simulink model "PWMGenerationComponent"  (R2026a)
settings: Solver=FixedStepDiscrete
settings Model: DataDictionary=TractionEmotorSoftwareArchInterfaceData.sldd  Creator=dakaihu  LastModifiedBy=dakaihu

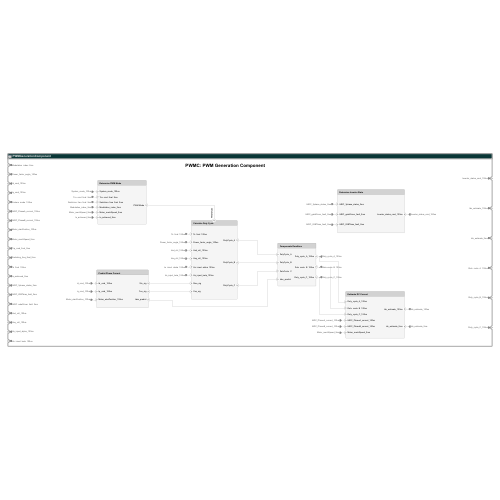
[thumbnail: Simulink's stored preview of the top-level diagram]
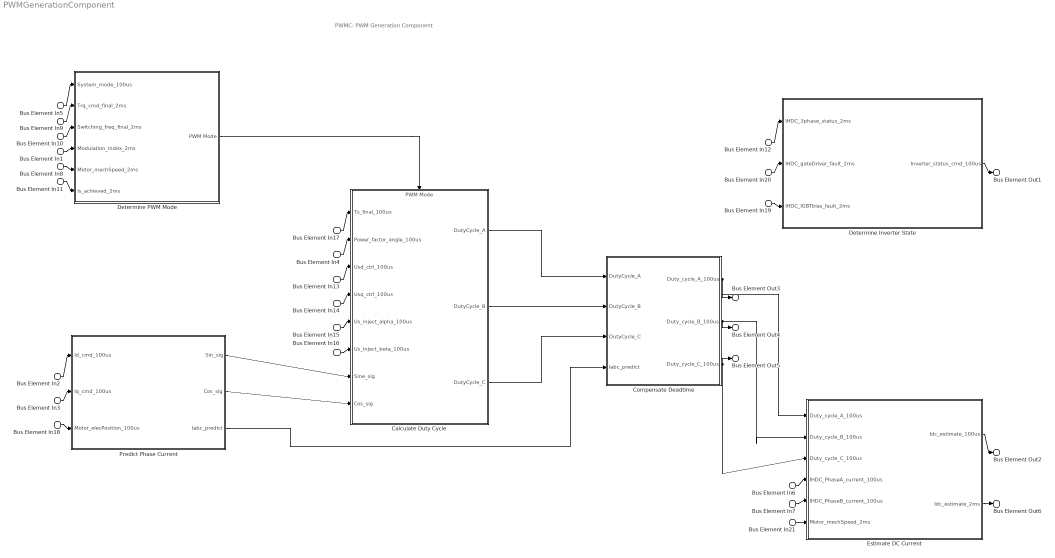
== system PWMGenerationComponent ==
  note: PWMC: PWM Generation Component
  Bus Element In1 : Inport  PortName=Modulation_index_2ms
  Bus Element In4 : Inport  Port=2  PortName=Power_factor_angle_100us
  Bus Element In2 : Inport  Port=3  PortName=Id_cmd_100us
  Bus Element In3 : Inport  Port=4  PortName=Iq_cmd_100us
  Bus Element In5 : Inport  Port=5  PortName=System_mode_100us
  Bus Element In6 : Inport  Port=6  PortName=IHDC_PhaseA_current_100us
  Bus Element In7 : Inport  Port=7  PortName=IHDC_PhaseB_current_100us
  Bus Element In18 : Inport  Port=8  PortName=Motor_elecPosition_100us
  Bus Element In8 : Inport  Port=9  PortName=Motor_mechSpeed_2ms
  Bus Element In21 : Inport  Port=9  PortName=Motor_mechSpeed_2ms
  Bus Element In9 : Inport  Port=10  PortName=Trq_cmd_final_2ms
  Bus Element In10 : Inport  Port=11  PortName=Switching_freq_final_2ms
  Bus Element In17 : Inport  Port=12  PortName=Ts_final_100us
  Bus Element In11 : Inport  Port=13  PortName=Is_achieved_2ms
  Bus Element In12 : Inport  Port=14  PortName=IHDC_3phase_status_2ms
  Bus Element In19 : Inport  Port=15  PortName=IHDC_IGBTbias_fault_2ms
  Bus Element In20 : Inport  Port=16  PortName=IHDC_gateDriver_fault_2ms
  Bus Element In13 : Inport  Port=17  PortName=Usd_ctrl_100us
  Bus Element In14 : Inport  Port=18  PortName=Usq_ctrl_100us
  Bus Element In15 : Inport  Port=19  PortName=Us_inject_alpha_100us
  Bus Element In16 : Inport  Port=20  PortName=Us_inject_beta_100us
  Calculate Duty Cycle : Subsystem
      settings: PortSchema="{\"entries\":[{\"content\":{\"headerSize\":26,\"margin\":15,\"minimumSpacing\":25,\"sides\":[{\"content\":{\"connectorIds\":[\"In2\",\"In3\",\"In4\",\"In5\",\"In6\",\"In7\",\"In8\",\"In9\"]},\"type\":\"ConnectorPlacement.EquallySpacedRectSide\",\"uuid\":\"a0c63ab2-75fe-4bec-b2b0-6e2e00a1a5a4\"},{\"content\":{\"connectorIds\":[\"Out1\",\"Out2\",\"Out3\"],\"side\":\"RIGHT\"},\"type\":\"ConnectorPlacement.EquallySpacedRectSide\",\"uuid\":\"05d605ea-8968-4533-a01c-bf4aae5caa93\"},{\"content\":{\"connectorIds\":[\"In1\"],\"side\":\"TOP\"},\"type\":\"ConnectorPlacement.EquallySpacedRectSide\",\"uuid\":\"27167c69-3967-4107-acce-f317c3d854af\"}]},\"type\":\"ConnectorPlacement.EquallySpacedConnector\",\"uuid\":\"c4d90da2-0f2a-4c00-bd24-85fead00d18f\"}],\"packageUris\":[\"http://schema.mathworks.com/mf0/Connector/R2020b\"],\"version\":\"1.0\"}"
  Compensate Deadtime : Subsystem
      settings: PortSchema="{\"entries\":[{\"content\":{\"headerSize\":26,\"margin\":15,\"minimumSpacing\":25,\"sides\":[{\"content\":{\"connectorIds\":[\"In1\",\"In2\",\"In3\",\"In4\"]},\"type\":\"ConnectorPlacement.EquallySpacedRectSide\",\"uuid\":\"a0c63ab2-75fe-4bec-b2b0-6e2e00a1a5a4\"},{\"content\":{\"connectorIds\":[\"Out1\",\"Out2\",\"Out3\"],\"side\":\"RIGHT\"},\"type\":\"ConnectorPlacement.EquallySpacedRectSide\",\"uuid\":\"05d605ea-8968-4533-a01c-bf4aae5caa93\"},{\"content\":{\"connectorIds\":[],\"side\":\"TOP\"},\"type\":\"ConnectorPlacement.EquallySpacedRectSide\",\"uuid\":\"27167c69-3967-4107-acce-f317c3d854af\"}]},\"type\":\"ConnectorPlacement.EquallySpacedConnector\",\"uuid\":\"c4d90da2-0f2a-4c00-bd24-85fead00d18f\"}],\"packageUris\":[\"http://schema.mathworks.com/mf0/Connector/R2020b\"],\"version\":\"1.0\"}"
  Determine Inverter State : Subsystem
      settings: PortSchema="{\"entries\":[{\"content\":{\"headerSize\":26,\"margin\":15,\"minimumSpacing\":25,\"sides\":[{\"content\":{\"connectorIds\":[\"In1\",\"In2\",\"In3\"]},\"type\":\"ConnectorPlacement.EquallySpacedRectSide\",\"uuid\":\"a0c63ab2-75fe-4bec-b2b0-6e2e00a1a5a4\"},{\"content\":{\"connectorIds\":[\"Out1\"],\"side\":\"RIGHT\"},\"type\":\"ConnectorPlacement.EquallySpacedRectSide\",\"uuid\":\"05d605ea-8968-4533-a01c-bf4aae5caa93\"},{\"content\":{\"connectorIds\":[],\"side\":\"TOP\"},\"type\":\"ConnectorPlacement.EquallySpacedRectSide\",\"uuid\":\"27167c69-3967-4107-acce-f317c3d854af\"}]},\"type\":\"ConnectorPlacement.EquallySpacedConnector\",\"uuid\":\"c4d90da2-0f2a-4c00-bd24-85fead00d18f\"}],\"packageUris\":[\"http://schema.mathworks.com/mf0/Connector/R2020b\"],\"version\":\"1.0\"}"
  Determine PWM Mode : Subsystem
      settings: PortSchema="{\"entries\":[{\"content\":{\"headerSize\":26,\"margin\":15,\"minimumSpacing\":25,\"sides\":[{\"content\":{\"connectorIds\":[\"In1\",\"In2\",\"In3\",\"In4\",\"In5\",\"In6\"]},\"type\":\"ConnectorPlacement.EquallySpacedRectSide\",\"uuid\":\"a0c63ab2-75fe-4bec-b2b0-6e2e00a1a5a4\"},{\"content\":{\"connectorIds\":[\"Out1\"],\"side\":\"RIGHT\"},\"type\":\"ConnectorPlacement.EquallySpacedRectSide\",\"uuid\":\"05d605ea-8968-4533-a01c-bf4aae5caa93\"},{\"content\":{\"connectorIds\":[],\"side\":\"TOP\"},\"type\":\"ConnectorPlacement.EquallySpacedRectSide\",\"uuid\":\"27167c69-3967-4107-acce-f317c3d854af\"}]},\"type\":\"ConnectorPlacement.EquallySpacedConnector\",\"uuid\":\"c4d90da2-0f2a-4c00-bd24-85fead00d18f\"}],\"packageUris\":[\"http://schema.mathworks.com/mf0/Connector/R2020b\"],\"version\":\"1.0\"}"
  Estimate DC Current : Subsystem
      settings: PortSchema="{\"entries\":[{\"content\":{\"headerSize\":26,\"margin\":15,\"minimumSpacing\":25,\"sides\":[{\"content\":{\"connectorIds\":[\"In1\",\"In2\",\"In3\",\"In4\",\"In5\",\"In6\"]},\"type\":\"ConnectorPlacement.EquallySpacedRectSide\",\"uuid\":\"a0c63ab2-75fe-4bec-b2b0-6e2e00a1a5a4\"},{\"content\":{\"connectorIds\":[\"Out1\",\"Out2\"],\"side\":\"RIGHT\"},\"type\":\"ConnectorPlacement.EquallySpacedRectSide\",\"uuid\":\"05d605ea-8968-4533-a01c-bf4aae5caa93\"},{\"content\":{\"connectorIds\":[],\"side\":\"TOP\"},\"type\":\"ConnectorPlacement.EquallySpacedRectSide\",\"uuid\":\"27167c69-3967-4107-acce-f317c3d854af\"}]},\"type\":\"ConnectorPlacement.EquallySpacedConnector\",\"uuid\":\"c4d90da2-0f2a-4c00-bd24-85fead00d18f\"}],\"packageUris\":[\"http://schema.mathworks.com/mf0/Connector/R2020b\"],\"version\":\"1.0\"}"
  Predict Phase Current : Subsystem
      settings: PortSchema="{\"entries\":[{\"content\":{\"headerSize\":26,\"margin\":15,\"minimumSpacing\":25,\"sides\":[{\"content\":{\"connectorIds\":[\"In1\",\"In2\",\"In3\"]},\"type\":\"ConnectorPlacement.EquallySpacedRectSide\",\"uuid\":\"a0c63ab2-75fe-4bec-b2b0-6e2e00a1a5a4\"},{\"content\":{\"connectorIds\":[\"Out1\",\"Out2\",\"Out3\"],\"side\":\"RIGHT\"},\"type\":\"ConnectorPlacement.EquallySpacedRectSide\",\"uuid\":\"05d605ea-8968-4533-a01c-bf4aae5caa93\"},{\"content\":{\"connectorIds\":[],\"side\":\"TOP\"},\"type\":\"ConnectorPlacement.EquallySpacedRectSide\",\"uuid\":\"27167c69-3967-4107-acce-f317c3d854af\"}]},\"type\":\"ConnectorPlacement.EquallySpacedConnector\",\"uuid\":\"c4d90da2-0f2a-4c00-bd24-85fead00d18f\"}],\"packageUris\":[\"http://schema.mathworks.com/mf0/Connector/R2020b\"],\"version\":\"1.0\"}"
  Bus Element Out1 : Outport  PortName=Inverter_status_cmd_100us
  Bus Element Out2 : Outport  Port=2  PortName=Idc_estimate_100us
  Bus Element Out6 : Outport  Port=3  PortName=Idc_estimate_2ms
  Bus Element Out3 : Outport  Port=4  PortName=Duty_cycle_A_100us
  Bus Element Out4 : Outport  Port=5  PortName=Duty_cycle_B_100us
  Bus Element Out5 : Outport  Port=6  PortName=Duty_cycle_C_100us
  wires:
  Bus Element In12/1 -> Determine Inverter State/1(IHDC_3phase_status_2ms)
  Bus Element In20/1 -> Determine Inverter State/2(IHDC_gateDriver_fault_2ms)
  Bus Element In19/1 -> Determine Inverter State/3(IHDC_IGBTbias_fault_2ms)
  Bus Element In2/1 -> Predict Phase Current/1(Id_cmd_100us)
  Bus Element In3/1 -> Predict Phase Current/2(Iq_cmd_100us)
  Bus Element In18/1 -> Predict Phase Current/3(Motor_elecPosition_100us)
  Predict Phase Current/3(Iabc_predict) -> Compensate Deadtime/4(Iabc_predict)
  Predict Phase Current/1(Sin_sig) -> Calculate Duty Cycle/8(Sine_sig)
  Predict Phase Current/2(Cos_sig) -> Calculate Duty Cycle/9(Cos_sig)
  Bus Element In13/1 -> Calculate Duty Cycle/4(Usd_ctrl_100us)
  Bus Element In14/1 -> Calculate Duty Cycle/5(Usq_ctrl_100us)
  Bus Element In15/1 -> Calculate Duty Cycle/6(Us_inject_alpha_100us)
  Bus Element In16/1 -> Calculate Duty Cycle/7(Us_inject_beta_100us)
  Bus Element In4/1 -> Calculate Duty Cycle/3(Power_factor_angle_100us)
  Bus Element In17/1 -> Calculate Duty Cycle/2(Ts_final_100us)
  Bus Element In5/1 -> Determine PWM Mode/1(System_mode_100us)
  Bus Element In9/1 -> Determine PWM Mode/2(Trq_cmd_final_2ms)
  Bus Element In1/1 -> Determine PWM Mode/4(Modulation_index_2ms)
  Bus Element In10/1 -> Determine PWM Mode/3(Switching_freq_final_2ms)
  Bus Element In8/1 -> Determine PWM Mode/5(Motor_mechSpeed_2ms)
  Bus Element In11/1 -> Determine PWM Mode/6(Is_achieved_2ms)
  Determine PWM Mode/1(PWM Mode) -> Calculate Duty Cycle/1(PWM Mode)
  Calculate Duty Cycle/1(DutyCycle_A) -> Compensate Deadtime/1(DutyCycle_A)
  Calculate Duty Cycle/2(DutyCycle_B) -> Compensate Deadtime/2(DutyCycle_B)
  Calculate Duty Cycle/3(DutyCycle_C) -> Compensate Deadtime/3(DutyCycle_C)
  Bus Element In6/1 -> Estimate DC Current/4(IHDC_PhaseA_current_100us)
  Bus Element In7/1 -> Estimate DC Current/5(IHDC_PhaseB_current_100us)
  Bus Element In21/1 -> Estimate DC Current/6(Motor_mechSpeed_2ms)
  Estimate DC Current/1(Idc_estimate_100us) -> Bus Element Out2/1
  Compensate Deadtime/1(Duty_cycle_A_100us) -> Bus Element Out3/1, Estimate DC Current/1(Duty_cycle_A_100us)
  Compensate Deadtime/2(Duty_cycle_B_100us) -> Bus Element Out4/1, Estimate DC Current/2(Duty_cycle_B_100us)
  Compensate Deadtime/3(Duty_cycle_C_100us) -> Bus Element Out5/1, Estimate DC Current/3(Duty_cycle_C_100us)
  Estimate DC Current/2(Idc_estimate_2ms) -> Bus Element Out6/1
  Determine Inverter State/1(Inverter_status_cmd_100us) -> Bus Element Out1/1

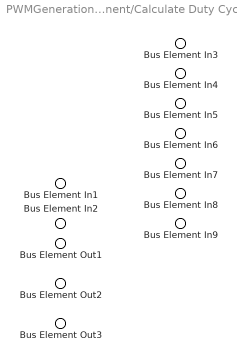
== system PWMGenerationComponent/Calculate Duty Cycle ==
  Bus Element In9 : Inport  PortName=PWM Mode
  Bus Element In8 : Inport  Port=2  PortName=Ts_final_100us
  Bus Element In7 : Inport  Port=3  PortName=Power_factor_angle_100us
  Bus Element In3 : Inport  Port=4  PortName=Usd_ctrl_100us
  Bus Element In4 : Inport  Port=5  PortName=Usq_ctrl_100us
  Bus Element In5 : Inport  Port=6  PortName=Us_inject_alpha_100us
  Bus Element In6 : Inport  Port=7  PortName=Us_inject_beta_100us
  Bus Element In1 : Inport  Port=8  PortName=Sine_sig
  Bus Element In2 : Inport  Port=9  PortName=Cos_sig
  Bus Element Out1 : Outport  PortName=DutyCycle_A
  Bus Element Out2 : Outport  Port=2  PortName=DutyCycle_B
  Bus Element Out3 : Outport  Port=3  PortName=DutyCycle_C

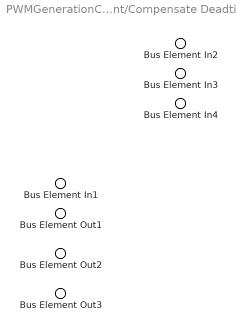
== system PWMGenerationComponent/Compensate Deadtime ==
  Bus Element In2 : Inport  PortName=DutyCycle_A
  Bus Element In3 : Inport  Port=2  PortName=DutyCycle_B
  Bus Element In4 : Inport  Port=3  PortName=DutyCycle_C
  Bus Element In1 : Inport  Port=4  PortName=Iabc_predict
  Bus Element Out1 : Outport  PortName=Duty_cycle_A_100us
  Bus Element Out2 : Outport  Port=2  PortName=Duty_cycle_B_100us
  Bus Element Out3 : Outport  Port=3  PortName=Duty_cycle_C_100us

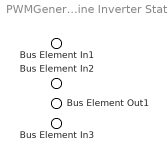
== system PWMGenerationComponent/Determine Inverter State ==
  Bus Element In1 : Inport  PortName=IHDC_3phase_status_2ms
  Bus Element In2 : Inport  Port=2  PortName=IHDC_gateDriver_fault_2ms
  Bus Element In3 : Inport  Port=3  PortName=IHDC_IGBTbias_fault_2ms
  Bus Element Out1 : Outport  PortName=Inverter_status_cmd_100us

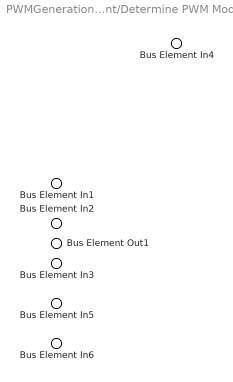
== system PWMGenerationComponent/Determine PWM Mode ==
  Bus Element In1 : Inport  PortName=System_mode_100us
  Bus Element In2 : Inport  Port=2  PortName=Trq_cmd_final_2ms
  Bus Element In4 : Inport  Port=3  PortName=Switching_freq_final_2ms
  Bus Element In3 : Inport  Port=4  PortName=Modulation_index_2ms
  Bus Element In5 : Inport  Port=5  PortName=Motor_mechSpeed_2ms
  Bus Element In6 : Inport  Port=6  PortName=Is_achieved_2ms
  Bus Element Out1 : Outport  PortName=PWM Mode

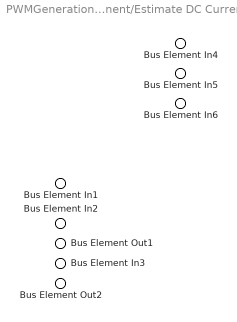
== system PWMGenerationComponent/Estimate DC Current ==
  Bus Element In4 : Inport  PortName=Duty_cycle_A_100us
  Bus Element In5 : Inport  Port=2  PortName=Duty_cycle_B_100us
  Bus Element In6 : Inport  Port=3  PortName=Duty_cycle_C_100us
  Bus Element In1 : Inport  Port=4  PortName=IHDC_PhaseA_current_100us
  Bus Element In2 : Inport  Port=5  PortName=IHDC_PhaseB_current_100us
  Bus Element In3 : Inport  Port=6  PortName=Motor_mechSpeed_2ms
  Bus Element Out1 : Outport  PortName=Idc_estimate_100us
  Bus Element Out2 : Outport  Port=2  PortName=Idc_estimate_2ms

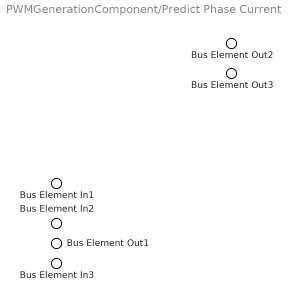
== system PWMGenerationComponent/Predict Phase Current ==
  Bus Element In1 : Inport  PortName=Id_cmd_100us
  Bus Element In2 : Inport  Port=2  PortName=Iq_cmd_100us
  Bus Element In3 : Inport  Port=3  PortName=Motor_elecPosition_100us
  Bus Element Out2 : Outport  PortName=Sin_sig
  Bus Element Out3 : Outport  Port=2  PortName=Cos_sig
  Bus Element Out1 : Outport  Port=3  PortName=Iabc_predict
